simulink model "exercise1"  (Simulink 7.1)
settings: Solver=ode45  StartTime=0.0  StopTime=10.0  RelTol=1e-3
values from neighbouring files (symbols this model uses):
  a = 1    [exercise1_script.m]
  b = 2    [exercise1_script.m]
settings Model: Creator=minyan09  LastModifiedBy=minyan09
settings DataIOCC: ExternalInput=[a, b]  InitialState=x(0)  SaveOutput=off  SaveState=on  SignalLogging=off

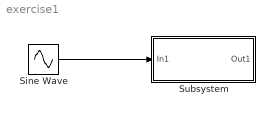
== system exercise1 ==
  Sine Wave : Sin  Bias=a  Frequency=b  SampleTime=0
  Subsystem : Subsystem
  wires:
  Sine Wave/1 -> Subsystem/1(In1)

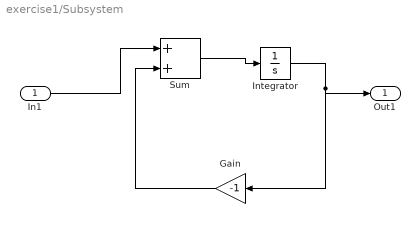
== system exercise1/Subsystem ==
  In1 : Inport  OutDataType=sfix(16)  OutScaling=2^0
  Gain : Gain  Orientation=left  Gain=-1  ParameterDataType=sfix(16)  ParameterScaling=2^0  OutDataType=sfix(16)  OutScaling=2^0
  Integrator : Integrator  InitialCondition=2
  Sum : Sum  Inputs=|++  OutDataType=sfix(16)  OutScaling=2^0
  Out1 : Outport  OutDataType=sfix(16)  OutScaling=2^0
  wires:
  In1/1 -> Sum/1
  Sum/1 -> Integrator/1
  Integrator/1 -> Out1/1, Gain/1
  Gain/1 -> Sum/2
